simulink model "OFDM"  (R2016a)
settings: Solver=VariableStepAuto  StartTime=0.0  StopTime=1  RelTol=1e-3
libraries: dspxfrm3 x5, dspmtrx3 x5, commdigbbndpm3 x3, commchan3 x2, commsink2 x2, commrandsrc2 x2
settings Model: Creator=dell  LastModifiedBy=dell

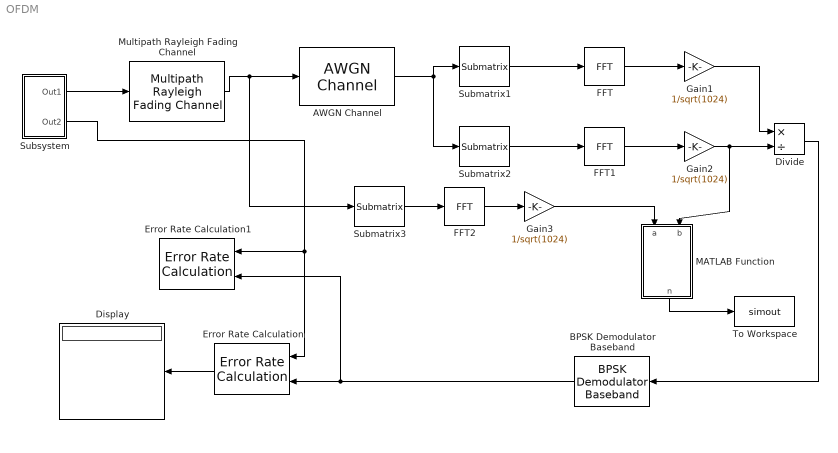
== system OFDM ==
  AWGN Channel : commchan3/AWGN Channel  InputProcessing=Columns as channels (frame based)  seed=67  noiseMode="Signal to noise ratio  (SNR)"  EbNodB=10  EsNodB=10  SNRdB=snr  bitsPerSym=1  Ps=1  Tsym=1  variance=1
  BPSK Demodulator Baseband : commdigbbndpm3/BPSK Demodulator Baseband  DecType=Hard decision  VarSource=Dialog  Variance=1  Ph=0  outDtype=Inherit via internal rule  derotateFactorWordLen=16  derotateFactorDataTypeStr=Inherit: Same word length as input  derotateFactorLastDataTypeStr=Inherit: Same word length as input
  Display : Display
  Divide : Product  Inputs=*/
  Error Rate Calculation : commsink2/Error Rate Calculation  N=0  st_delay=0  cp_mode=Entire frame  subframe=[]  PMode=Port  WsName=ErrorVec  RsMode2=off  stop=off  numErr=100  maxBits=1e6
  Error Rate Calculation1 : commsink2/Error Rate Calculation  N=0  st_delay=0  cp_mode=Entire frame  subframe=[]  PMode=Workspace  WsName=ErrorVec  RsMode2=off  stop=off  numErr=100  maxBits=1e6
  FFT : dspxfrm3/FFT  FFTImplementation=Auto  CompMethod=Table lookup  TableOpt=NEW  TableOptActive=Speed  BitRevOrder=off  Normalize=off  InheritFFTLength=on  FFTLength=64  WrapInput=on  roundingMode=Floor  overflowMode=off  firstCoeffDataTypeStr=Inherit: Same word length as input  firstCoeffLastDataTypeStr=Inherit: Same word length as input  outputMin=[]  outputMax=[]
  FFT1 : dspxfrm3/FFT  FFTImplementation=Auto  CompMethod=Table lookup  TableOpt=NEW  TableOptActive=Speed  BitRevOrder=off  Normalize=off  InheritFFTLength=on  FFTLength=64  WrapInput=on  roundingMode=Floor  overflowMode=off  firstCoeffDataTypeStr=Inherit: Same word length as input  firstCoeffLastDataTypeStr=Inherit: Same word length as input  outputMin=[]  outputMax=[]
  FFT2 : dspxfrm3/FFT  FFTImplementation=Auto  CompMethod=Table lookup  TableOpt=NEW  TableOptActive=Speed  BitRevOrder=off  Normalize=off  InheritFFTLength=on  FFTLength=64  WrapInput=on  roundingMode=Floor  overflowMode=off  firstCoeffDataTypeStr=Inherit: Same word length as input  firstCoeffLastDataTypeStr=Inherit: Same word length as input  outputMin=[]  outputMax=[]
  Gain1 : Gain  Gain=1/sqrt(1024)
  Gain2 : Gain  Gain=1/sqrt(1024)
  Gain3 : Gain  Gain=1/sqrt(1024)
  MATLAB Function : MATLAB Function  TreatAsAtomicUnit=on
  Multipath Rayleigh Fading Channel : commchan3/Multipath Rayleigh Fading Channel  maxDopplerShift=40  spectrumType=Jakes  sigmaGaussian=1/sqrt(2)  coeffRounded=[1 -1.72 0.785]  freqMinMaxRJakes=[0 1]  freqMinMaxAJakes=[0 1]  sigmaGaussian1=1/sqrt(2)  sigmaGaussian2=1/sqrt(2)  centerFreqGaussian1=0.0  centerFreqGaussian2=0.0  gainGaussian1=0.5  gainGaussian2=0.5  coeffBell=9  dopplerSpectrum=doppler.jakes  pathDelays=[0 2e-6 3e-6]  avgPathGaindB=[0 -3 -6]  normalizePathGains=on  seed=73  enableProbe=0  openVisAtStart=off  outPathGains=off  outDelay=off
  Submatrix1 : dspmtrx3/Submatrix  RowSpan=Range of rows  RowStartMode=Index  RowStartIndex=1280+256+1  RowEndMode=Last  RowEndIndex=1  ColSpan=Range of columns  ColStartMode=First  ColStartIndex=1  ColEndMode=Last  ColEndIndex=1
  Submatrix2 : dspmtrx3/Submatrix  RowSpan=Range of rows  RowStartMode=Index  RowStartIndex=256+1  RowEndMode=Index  RowEndIndex=1280  ColSpan=Range of columns  ColStartMode=First  ColStartIndex=1  ColEndMode=Last  ColEndIndex=1
  Submatrix3 : dspmtrx3/Submatrix  RowSpan=Range of rows  RowStartMode=Index  RowStartIndex=256+1  RowEndMode=Index  RowEndIndex=1280  ColSpan=Range of columns  ColStartMode=First  ColStartIndex=1  ColEndMode=Last  ColEndIndex=1
  Subsystem : Subsystem
  To Workspace : ToWorkspace  VariableName=simout  SampleTime=-1
  wires:
  Multipath Rayleigh Fading Channel/1 -> Submatrix3/1, AWGN Channel/1
  Submatrix1/1 -> FFT/1
  FFT/1 -> Gain1/1
  Divide/1 -> BPSK Demodulator Baseband/1
  BPSK Demodulator Baseband/1 -> Error Rate Calculation1/2, Error Rate Calculation/2
  Error Rate Calculation/1 -> Display/1
  Subsystem/1(Out1) -> Multipath Rayleigh Fading Channel/1
  Subsystem/2(Out2) -> Error Rate Calculation1/1, Error Rate Calculation/1
  Gain1/1 -> Divide/1
  Submatrix2/1 -> FFT1/1
  FFT1/1 -> Gain2/1
  Gain2/1 -> MATLAB Function/2(b), Divide/2
  AWGN Channel/1 -> Submatrix2/1, Submatrix1/1
  MATLAB Function/1(n) -> To Workspace/1
  Submatrix3/1 -> FFT2/1
  FFT2/1 -> Gain3/1
  Gain3/1 -> MATLAB Function/1(a)

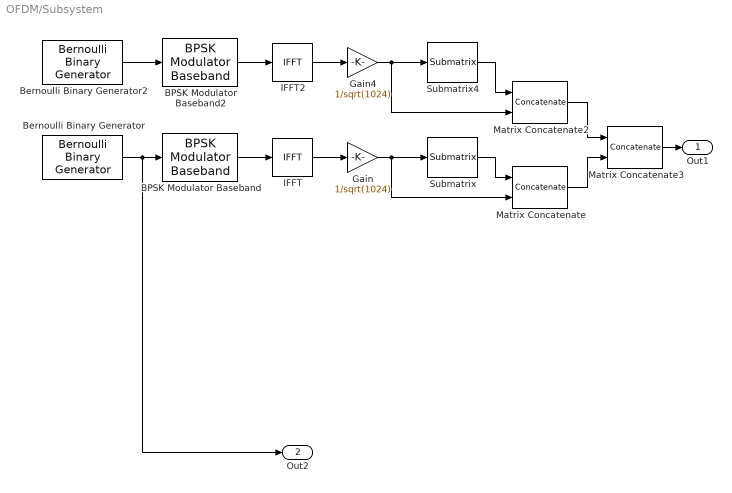
== system OFDM/Subsystem ==
  BPSK Modulator Baseband : commdigbbndpm3/BPSK Modulator Baseband  Ph=0  outDtype=double  outWordLen=16  outUDDataType=sfix(16)  outFracLenMode=Best precision  outFracLen=15  outDataTypeStr=double  outLastDataTypeStr=double
  BPSK Modulator Baseband2 : commdigbbndpm3/BPSK Modulator Baseband  Ph=0  outDtype=double  outWordLen=16  outUDDataType=sfix(16)  outFracLenMode=Best precision  outFracLen=15  outDataTypeStr=double  outLastDataTypeStr=double
  Bernoulli Binary Generator : commrandsrc2/Bernoulli Binary Generator  P=0.5  seed=61  Ts=1e-7  frameBased=on  sampPerFrame=1024  orient=off  outDataType=double
  Bernoulli Binary Generator2 : commrandsrc2/Bernoulli Binary Generator  P=1  seed=61  Ts=1e-7  frameBased=on  sampPerFrame=1024  orient=off  outDataType=double
  Gain : Gain  Gain=1/sqrt(1024)
  Gain4 : Gain  Gain=1/sqrt(1024)
  IFFT : dspxfrm3/IFFT  FFTImplementation=Auto  CompMethod=Table lookup  TableOpt=NEW  TableOptActive=Speed  BitRevOrder=off  cs_in=off  Normalize=off  InheritFFTLength=on  FFTLength=64  WrapInput=on  mode=Complex  outSamplingMode=Frame based  roundingMode=Floor  overflowMode=off  firstCoeffDataTypeStr=Inherit: Same word length as input  firstCoeffLastDataTypeStr=Inherit: Same word length as input  outputMin=[]  outputMax=[]
  IFFT2 : dspxfrm3/IFFT  FFTImplementation=Auto  CompMethod=Table lookup  TableOpt=NEW  TableOptActive=Speed  BitRevOrder=off  cs_in=off  Normalize=off  InheritFFTLength=on  FFTLength=64  WrapInput=on  mode=Complex  outSamplingMode=Frame based  roundingMode=Floor  overflowMode=off  firstCoeffDataTypeStr=Inherit: Same word length as input  firstCoeffLastDataTypeStr=Inherit: Same word length as input  outputMin=[]  outputMax=[]
  Matrix Concatenate : Concatenate  Mode=Multidimensional array
  Matrix Concatenate2 : Concatenate  Mode=Multidimensional array
  Matrix Concatenate3 : Concatenate  Mode=Multidimensional array
  Submatrix : dspmtrx3/Submatrix  RowSpan=Range of rows  RowStartMode=Index  RowStartIndex=1024-256+1  RowEndMode=Last  RowEndIndex=1  ColSpan=Range of columns  ColStartMode=First  ColStartIndex=1  ColEndMode=Last  ColEndIndex=1
  Submatrix4 : dspmtrx3/Submatrix  RowSpan=Range of rows  RowStartMode=Index  RowStartIndex=1024-256+1  RowEndMode=Last  RowEndIndex=1  ColSpan=Range of columns  ColStartMode=First  ColStartIndex=1  ColEndMode=Last  ColEndIndex=1
  Out1 : Outport
  Out2 : Outport  Port=2
  wires:
  Bernoulli Binary Generator/1 -> Out2/1, BPSK Modulator Baseband/1
  Submatrix/1 -> Matrix Concatenate/1
  IFFT2/1 -> Gain4/1
  BPSK Modulator Baseband2/1 -> IFFT2/1
  Bernoulli Binary Generator2/1 -> BPSK Modulator Baseband2/1
  Gain4/1 -> Matrix Concatenate2/2, Submatrix4/1
  Submatrix4/1 -> Matrix Concatenate2/1
  Matrix Concatenate2/1 -> Matrix Concatenate3/1
  Matrix Concatenate/1 -> Matrix Concatenate3/2
  Matrix Concatenate3/1 -> Out1/1
  Gain/1 -> Matrix Concatenate/2, Submatrix/1
  BPSK Modulator Baseband/1 -> IFFT/1
  IFFT/1 -> Gain/1

== matlab function OFDM/MATLAB Function ==
  data: a input; n output; b input
function n= mse(a,b)
%#codegen

n=sum(abs(a-b).^2)/sum(abs(a).^2);
